simulink model "DCmotor_control_diagram"  (R2021a)
settings: Solver=VariableStepAuto  StartTime=0.0  StopTime=5  RelTol=1e-3
values from neighbouring files (symbols this model uses):
  J = 465.8e-7    (= 4.658e-05)    [power_brushlessDCmotor_moog2328_control_scheme.m]
undefined symbols (not defined in the file or in its folder): Ir, Ke, Kt, L, Mmax, R
libraries: pid_lib x1
settings Model: Creator=Admin  LastModifiedBy=marin
settings SolverCC: AlgebraicLoopSolver=TrustRegion
settings DataIOCC: ReturnWorkspaceOutputs=off
settings DebuggingCC: SFMachineParentedDataDiag=warning  ArithmeticOperatorsInVariantConditions=warning
settings SFSimCC: SimUseLocalCustomCode=off  CustomCodeUndefinedFunction=UseInterfaceOnly
settings RTWCC: RTWUseLocalCustomCode=off
settings CodeAppCC: StateflowObjectComments=on

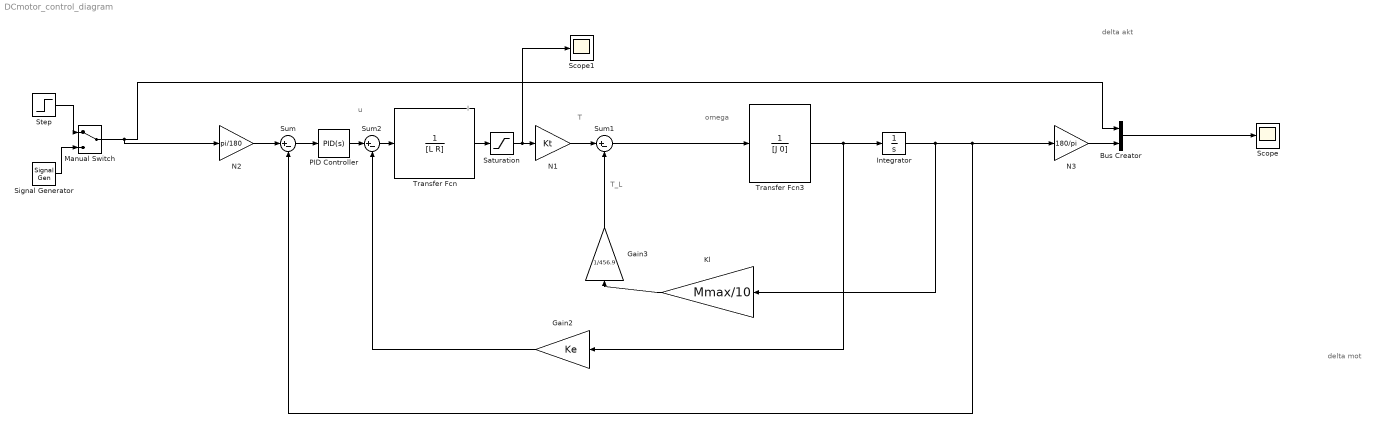
== system DCmotor_control_diagram ==
  note: T_L
  note: delta akt
  note: delta mot
  note: omega
  note: T
  note: I
  note: u
  Bus Creator : BusCreator  Inputs=2
  Gain2 : Gain  Gain=Ke
  Gain3 : Gain  Gain=1/456.9
  Integrator : Integrator
  Kl : Gain  Gain=Mmax/10
  Manual Switch : ManualSwitch
  N1 : Gain  Gain=Kt
  N2 : Gain  Gain=pi/180
  N3 : Gain  Gain=180/pi
  PID Controller : pid_lib/PID Controller  Controller=PID  Form=Parallel  TimeDomain=Continuous-time  UseExternalTs=off  SampleTime=-1  IntegratorMethod=Forward Euler  FilterMethod=Forward Euler  ControllerParametersSource=internal  P=1.97984715541991  I=27.0082733381866  D=0.0105535523473669  UseFilter=on  N=104.923127808584  TunerSelectOption=Transfer Function Based (PID Tuner App)  InitialConditionSource=internal  InitialConditionForIntegrator=0  InitialConditionForFilter=0  DifferentiatorICPrevScaledInput=0  ExternalReset=none  TrackingMode=off  Kt=1  LimitOutput=off  SatLimitsSource=internal  UpperSaturationLimit=inf  LowerSaturationLimit=-inf  LinearizeAsGain=on  AntiWindupMode=none  Kb=1  POutMin=[]  POutMax=[]  IOutMin=[]  IOutMax=[]  DOutMin=[]  DOutMax=[]  NOutMin=[]  NOutMax=[]  SumOutMin=[]  SumOutMax=[]  SaturationOutMin=[]  SaturationOutMax=[]  PParamMin=[]  PParamMax=[]  IParamMin=[]  IParamMax=[]  DParamMin=[]  DParamMax=[]  NParamMin=[]  NParamMax=[]  KbParamMin=[]  KbParamMax=[]  KtParamMin=[]  KtParamMax=[]  KbOutMin=[]  KbOutMax=[]  KtOutMin=[]  KtOutMax=[]  IntegratorOutMin=[]  IntegratorOutMax=[]  FilterOutMin=[]  FilterOutMax=[]  SumI1OutMin=[]  SumI1OutMax=[]  SumI2OutMin=[]  SumI2OutMax=[]  SumI3OutMin=[]  SumI3OutMax=[]  SumI4OutMin=[]  SumI4OutMax=[]  SumDOutMin=[]  SumDOutMax=[]  DifferentiatorOutMin=[]  DifferentiatorOutMax=[]  FilterDiffOutCoefMin=[]  FilterDiffOutCoefMax=[]  ReciprocalOutMin=[]  ReciprocalOutMax=[]  SumDenOutMin=[]  SumDenOutMax=[]  SumNumOutMin=[]  SumNumOutMax=[]  DivideOutMin=[]  DivideOutMax=[]  UdiffTsProdOutMin=[]  UdiffTsProdOutMax=[]  NTsProdOutMin=[]  NTsProdOutMax=[]  UintegralTsProdOutMin=[]  UintegralTsProdOutMax=[]  UngainTsProdOutMin=[]  UngainTsProdOutMax=[]  IntegratorContinuousStateAttributes=''  IntegratorStateMustResolveToSignalObject=off  IntegratorRTWStateStorageClass=Auto  FilterContinuousStateAttributes=''  FilterStateMustResolveToSignalObject=off  FilterRTWStateStorageClass=Auto  ParallelPVariant=InternalParameters  IdealPVariant=Disabled  IVariant=InternalParameters  DVariant=InternalParameters  IntegratorVariant=Continuous  SatVariant=Disabled  AWVariant=Passthrough  PCopyVariant=Disabled  TRVariant=Disabled  FdbkBlocksVariant=Forward  IdealPFdbkVariant=Disabled  SatFdbkVariant=Disabled  DerivativeFilterVariant=ContFilter  NVariant=InternalParameters  NCopyVariant=Disabled  FilterICVariant=InternalICsFilter  IntegratorICVariant=InternalICs  ExternalResetVariant=Disabled  TRSumVariant=Passthrough  SumFdbkVariant=Disabled  SumVariant=Sum_PID  TsampFilterVariant=InternalTs  TsampNgainVariant=Passthrough  TsampIntegralVariant=Passthrough  ExternalSaturationOutDataTypeStr=Inherit: Same as second input
  Saturation : Saturate  UpperLimit=Ir  LowerLimit=-Ir
  Scope : Scope
  Scope1 : Scope
  Signal Generator : SignalGenerator  Units=rad/sec
  Step : Step  After=10  SampleTime=0
  Sum : Sum  Inputs=|+-
  Sum1 : Sum  Inputs=|+-
  Sum2 : Sum  Inputs=|+-
  Transfer Fcn : TransferFcn  Denominator=[L R]
  Transfer Fcn3 : TransferFcn  Denominator=[J 0]
  wires:
  Sum/1 -> PID Controller/1
  Transfer Fcn/1 -> Saturation/1
  Sum1/1 -> Transfer Fcn3/1
  Transfer Fcn3/1 -> Gain2/1, Integrator/1
  Kl/1 -> Gain3/1
  Manual Switch/1 -> N2/1, Bus Creator/1
  PID Controller/1 -> Sum2/1
  Sum2/1 -> Transfer Fcn/1
  Saturation/1 -> Scope1/1, N1/1
  N1/1 -> Sum1/1
  Gain2/1 -> Sum2/2
  Step/1 -> Manual Switch/1
  Signal Generator/1 -> Manual Switch/2
  N2/1 -> Sum/1
  Gain3/1 -> Sum1/2
  N3/1 -> Bus Creator/2
  Bus Creator/1 -> Scope/1
  Integrator/1 -> Kl/1, Sum/2, N3/1
